simulink model "bus_create_blk"  (R2019a)
settings: Solver=VariableStepAuto  StartTime=0.0  StopTime=10.0  RelTol=1e-3
libraries: xbsIndex_r4 x7
settings Model: Creator=Ross Donnachie  LastModifiedBy=Ross Donnachie

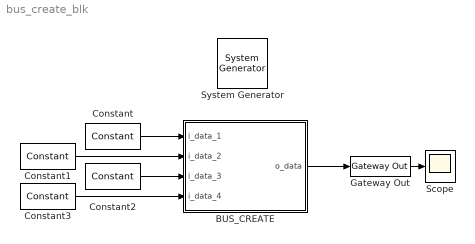
== system bus_create_blk ==
  " System Generator" : xbsIndex_r4/ System Generator  Tag=genX  xilinxfamily=kintex7  part=xc7k325t  speed=-3  package=fbg676  synthesis_tool=Vivado  clock_wrapper=Clock Enables  directory=./netlist  proj_type=Vivado  Synth_file=Vivado Synthesis Defaults  Impl_file=Vivado Implementation Defaults  testbench=off  simulink_period=1  sysclk_period=10  dcm_input_clock_period=10  incr_netlist=off  trim_vbits=Everywhere in SubSystem  dbl_ovrd=According to Block Masks  core_generation=According to Block Masks  run_coregen=off  deprecated_control=off  eval_field=0  block_type=sysgen
  BUS_CREATE : Subsystem  mask{bit_widths=4,1,2,1}
      mask prompts: bit_widths "Input bit-widths:"
      mask init:
      | Simulink.Block.eval([gcb, '/bus_create']);
      | 
      | bus_create_subsys2bb_knit();
      mask DialogControl DescTextVar Prompt: Creates a 'bus' from bit-vectors. The output will be the consequetive concatenation of each input, starting at the most significant bit.
  Constant : xbsIndex_r4/Constant  const=15  gui_display_data_type=Fixed-point  arith_type=Unsigned  n_bits=4  bin_pt=0  preci_type=Single  exp_width=8  frac_width=24  explicit_period=on  period=1  equ=P=C  opselect=C  inp2=PCIN>>17  opr=+  inp1=P  carry=CIN  dbl_ovrd=off  block_type=constant
  Constant1 : xbsIndex_r4/Constant  const=1.0  gui_display_data_type=Fixed-point  arith_type=Unsigned  n_bits=1  bin_pt=0  preci_type=Single  exp_width=8  frac_width=24  explicit_period=on  period=1  equ=P=C  opselect=C  inp2=PCIN>>17  opr=+  inp1=P  carry=CIN  dbl_ovrd=off  block_type=constant
  Constant2 : xbsIndex_r4/Constant  const=3  gui_display_data_type=Fixed-point  arith_type=Unsigned  n_bits=2  bin_pt=0  preci_type=Single  exp_width=8  frac_width=24  explicit_period=on  period=1  equ=P=C  opselect=C  inp2=PCIN>>17  opr=+  inp1=P  carry=CIN  dbl_ovrd=off  block_type=constant
  Constant3 : xbsIndex_r4/Constant  const=1  gui_display_data_type=Fixed-point  arith_type=Unsigned  n_bits=1  bin_pt=0  preci_type=Single  exp_width=8  frac_width=24  explicit_period=on  period=1  equ=P=C  opselect=C  inp2=PCIN>>17  opr=+  inp1=P  carry=CIN  dbl_ovrd=off  block_type=constant
  Gateway Out : xbsIndex_r4/Gateway Out  inherit_from_input=off  hdl_port=on  rows=1  columns=1  UseAsDAC=off  DACChannel='1'  interface=None  automatic_assignment=on  address_offset=hex2dec('00')  intf_name=''  intf_description=''  timing_constraint=None  locs_specified=off  LOCs={}  io_standard={}  block_type=gatewayout
  Scope : Scope
  wires:
  Constant/1 -> BUS_CREATE/1(i_data_1)
  Constant1/1 -> BUS_CREATE/2(i_data_2)
  Constant2/1 -> BUS_CREATE/3(i_data_3)
  Constant3/1 -> BUS_CREATE/4(i_data_4)
  BUS_CREATE/1(o_data) -> Gateway Out/1
  Gateway Out/1 -> Scope/1

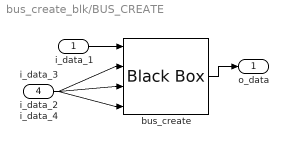
== system bus_create_blk/BUS_CREATE ==
  i_data_1 : Inport
  i_data_2 : Inport  Port=2
  i_data_3 : Inport  Port=3
  i_data_4 : Inport  Port=4
  bus_create : xbsIndex_r4/Black Box  init_code=bus_create_arbitrary_config  sim_method=ISE Simulator  verbose=on  block_type=blackbox2
  o_data : Outport
  wires:
  bus_create/1 -> o_data/1
  i_data_1/1 -> bus_create/1
  i_data_2/1 -> bus_create/2
  i_data_3/1 -> bus_create/3
  i_data_4/1 -> bus_create/4
